simulink model "cart_pendulum_nonlinear"  (R2024b)
settings: Solver=ode4  StartTime=0.0  StopTime=3  FixedStep=1e-5  MaxStep=0.001  RelTol=1e-3
values from neighbouring files (symbols this model uses):
  g = 9.81    [wheeled_balancer_model_simscape_script.m]
  J = (I_motor + I_bump + I_batt + I_cb)    (= 0.000441007536814)    [wheeled_balancer_model_simscape_script.m]
  l = .1    (= 0.1)    [Scratchwork_pendulums.m]    (also in wheeled_balancer_model_simscape_script.m = CM_rot)
  m = 1    [Scratchwork_pendulums.m]    (also in wheeled_balancer_model_simscape_script.m = 0.2983)
  m_c = (m_wheels)    (= 0.0397)    [wheeled_balancer_model_simscape_script.m]
  mu_c = 0.02    [wheeled_balancer_model_simscape_script.m]
  r = 0.01    [Scratchwork_pendulums.m]    (also in wheeled_balancer_model_simscape_script.m = 0.04)
  T = 1/100    (= 0.01)    [wheeled_balancer_model_simscape_script.m]
  theta_init = 0    [wheeled_balancer_model_simscape_script.m]
undefined symbols (not defined in the file or in its folder): Cd
settings Model: Creator=teowi  LastModifiedBy=teowi

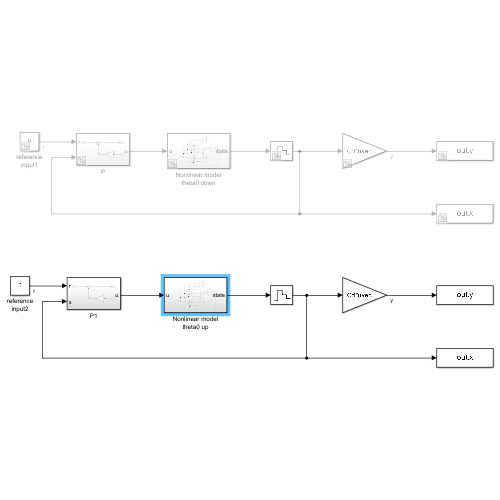
[thumbnail: Simulink's stored preview of the top-level diagram]
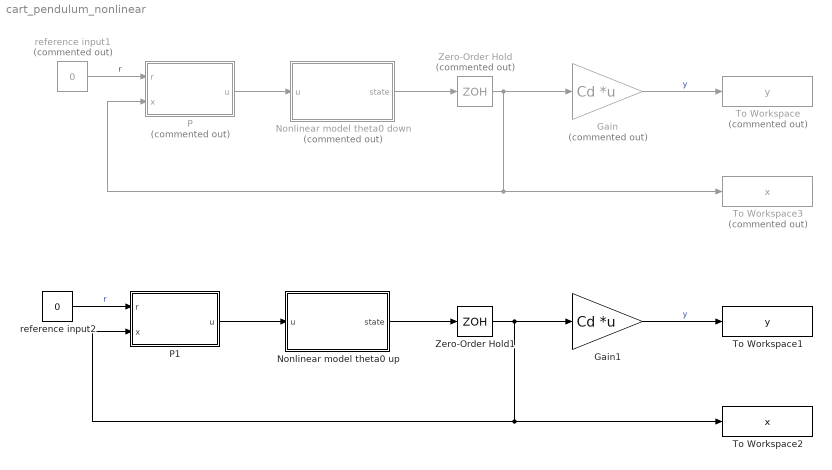
== system cart_pendulum_nonlinear ==
  Gain : Gain  Commented=on  Gain=Cd  Multiplication=Matrix(K*u) (u vector)
  Gain1 : Gain  Gain=Cd  Multiplication=Matrix(K*u) (u vector)
  Nonlinear model theta0 down : Subsystem  Commented=on
  Nonlinear model theta0 up : Subsystem
  P : Subsystem  Commented=on
  P1 : Subsystem
  To Workspace : ToWorkspace  Commented=on  VariableName=y  SaveFormat=Timeseries  SampleTime=-1
  To Workspace1 : ToWorkspace  VariableName=y  SaveFormat=Timeseries  SampleTime=-1
  To Workspace2 : ToWorkspace  VariableName=x  SaveFormat=Timeseries  SampleTime=-1
  To Workspace3 : ToWorkspace  Commented=on  VariableName=x  SaveFormat=Timeseries  SampleTime=-1
  Zero-Order Hold : ZeroOrderHold  Commented=on  SampleTime=T
  Zero-Order Hold1 : ZeroOrderHold  SampleTime=T
  reference input1 : Constant  Commented=on  Value=0
  reference input2 : Constant  Value=0
  wires:
  Gain/1 -> To Workspace/1  "y"
  Zero-Order Hold/1 -> P/2(x), To Workspace3/1, Gain/1
  Nonlinear model theta0 down/1(state) -> Zero-Order Hold/1
  P/1(u) -> Nonlinear model theta0 down/1(u)
  reference input1/1 -> P/1(r)  "r"
  Gain1/1 -> To Workspace1/1  "y"
  Nonlinear model theta0 up/1(state) -> Zero-Order Hold1/1
  reference input2/1 -> P1/1(r)  "r"
  Zero-Order Hold1/1 -> P1/2(x), To Workspace2/1, Gain1/1
  P1/1(u) -> Nonlinear model theta0 up/1(u)

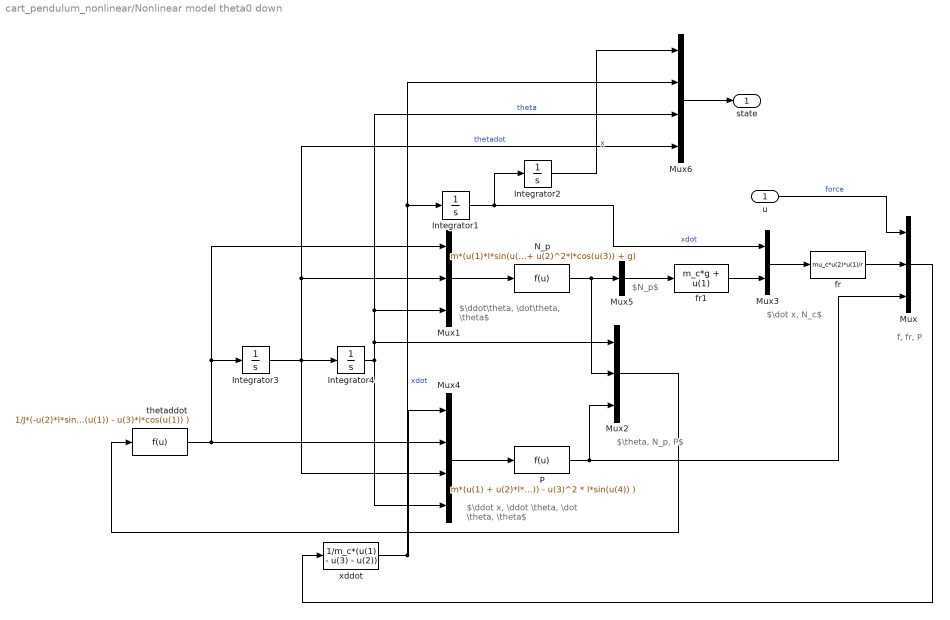
== system cart_pendulum_nonlinear/Nonlinear model theta0 down ==
  note: f, fr, P
  note: $\theta, N_p, P$
  note: $\dot x, N_c$
  note: $N_p$
  note: $\ddot\theta, \dot\theta, \theta$
  note: $\ddot x, \ddot \theta, \dot \theta, \theta$
  u : Inport
  Integrator1 : Integrator
  Integrator2 : Integrator
  Integrator3 : Integrator
  Integrator4 : Integrator  InitialCondition=theta_init
  Mux : Mux  Inputs=3
  Mux1 : Mux  Inputs=3
  Mux2 : Mux  Inputs=3
  Mux3 : Mux  Inputs=2
  Mux4 : Mux
  Mux5 : Mux  Inputs=1
  Mux6 : Mux
  N_p : Fcn  Expr=m*(u(1)*l*sin(u(3)) + u(2)^2*l*cos(u(3)) + g)
  P : Fcn  Expr=m*(u(1) + u(2)*l*cos(u(4)) - u(3)^2 * l*sin(u(4)) )
  fr : Fcn  Expr=mu_c*u(2)*u(1)/r
  fr1 : Fcn  Expr=m_c*g + u(1)
  thetaddot : Fcn  Expr=1/J*(-u(2)*l*sin(u(1)) - u(3)*l*cos(u(1)) )
  xddot : Fcn  Expr=1/m_c*(u(1) - u(3) - u(2))
  state : Outport
  wires:
  Mux2/1 -> thetaddot/1
  Integrator1/1 -> Integrator2/1, Mux3/1  "xdot"
  xddot/1 -> Mux6/2, Integrator1/1, Mux4/1  "xdot"
  thetaddot/1 -> Mux1/1, Integrator3/1, Mux4/2
  Integrator4/1 -> Mux2/1, Mux6/3, Mux1/3, Mux4/4  "theta"
  Integrator3/1 -> Mux4/3, Integrator4/1, Mux6/4, Mux1/2  "thetadot"
  Mux4/1 -> P/1
  Mux1/1 -> N_p/1
  N_p/1 -> Mux5/1, Mux2/2
  fr1/1 -> Mux3/2
  P/1 -> Mux/3, Mux2/3
  Mux5/1 -> fr1/1
  Mux/1 -> xddot/1
  Mux3/1 -> fr/1
  u/1 -> Mux/1  "force"
  fr/1 -> Mux/2
  Integrator2/1 -> Mux6/1  "x"
  Mux6/1 -> state/1

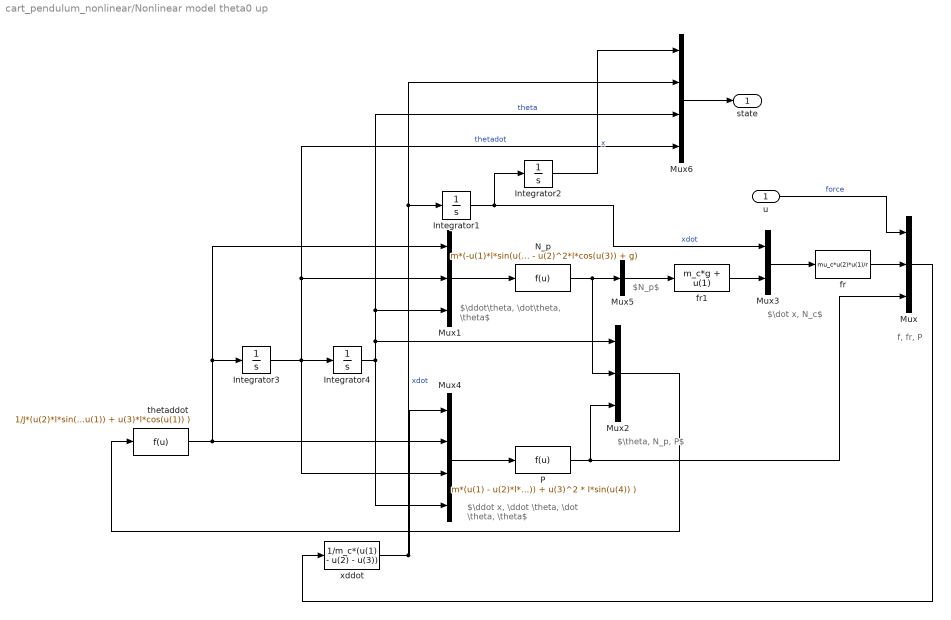
== system cart_pendulum_nonlinear/Nonlinear model theta0 up ==
  note: f, fr, P
  note: $\theta, N_p, P$
  note: $\dot x, N_c$
  note: $N_p$
  note: $\ddot\theta, \dot\theta, \theta$
  note: $\ddot x, \ddot \theta, \dot \theta, \theta$
  u : Inport
  Integrator1 : Integrator
  Integrator2 : Integrator
  Integrator3 : Integrator
  Integrator4 : Integrator  InitialCondition=theta_init
  Mux : Mux  Inputs=3
  Mux1 : Mux  Inputs=3
  Mux2 : Mux  Inputs=3
  Mux3 : Mux  Inputs=2
  Mux4 : Mux
  Mux5 : Mux  Inputs=1
  Mux6 : Mux
  N_p : Fcn  Expr=m*(-u(1)*l*sin(u(3)) - u(2)^2*l*cos(u(3)) + g)
  P : Fcn  Expr=m*(u(1) - u(2)*l*cos(u(4)) + u(3)^2 * l*sin(u(4)) )
  fr : Fcn  Expr=mu_c*u(2)*u(1)/r
  fr1 : Fcn  Expr=m_c*g + u(1)
  thetaddot : Fcn  Expr=1/J*(u(2)*l*sin(u(1)) + u(3)*l*cos(u(1)) )
  xddot : Fcn  Expr=1/m_c*(u(1) - u(2) - u(3))
  state : Outport
  wires:
  Mux2/1 -> thetaddot/1
  Integrator1/1 -> Integrator2/1, Mux3/1  "xdot"
  xddot/1 -> Mux6/2, Integrator1/1, Mux4/1  "xdot"
  thetaddot/1 -> Mux1/1, Integrator3/1, Mux4/2
  Integrator4/1 -> Mux2/1, Mux6/3, Mux1/3, Mux4/4  "theta"
  Integrator3/1 -> Mux4/3, Integrator4/1, Mux6/4, Mux1/2  "thetadot"
  Mux4/1 -> P/1
  Mux1/1 -> N_p/1
  N_p/1 -> Mux5/1, Mux2/2
  fr1/1 -> Mux3/2
  P/1 -> Mux/3, Mux2/3
  Mux5/1 -> fr1/1
  Mux/1 -> xddot/1
  Mux3/1 -> fr/1
  u/1 -> Mux/1  "force"
  fr/1 -> Mux/2
  Integrator2/1 -> Mux6/1  "x"
  Mux6/1 -> state/1

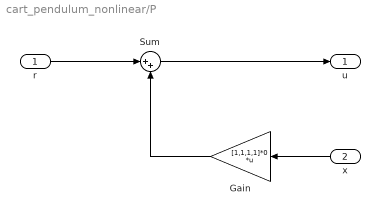
== system cart_pendulum_nonlinear/P ==
  r : Inport
  x : Inport  Port=2
  Gain : Gain  Gain=[1,1,1,1]*0  Multiplication=Matrix(K*u) (u vector)
  Sum : Sum  Inputs=|++
  u : Outport
  wires:
  r/1 -> Sum/1
  x/1 -> Gain/1
  Gain/1 -> Sum/2
  Sum/1 -> u/1

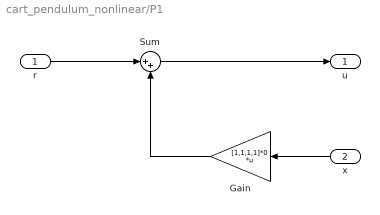
== system cart_pendulum_nonlinear/P1 ==
  r : Inport
  x : Inport  Port=2
  Gain : Gain  Gain=[1,1,1,1]*0  Multiplication=Matrix(K*u) (u vector)
  Sum : Sum  Inputs=|++
  u : Outport
  wires:
  r/1 -> Sum/1
  x/1 -> Gain/1
  Gain/1 -> Sum/2
  Sum/1 -> u/1
